simulink model "Neural_Network"  (R2013a)
settings: Solver=ode45  StartTime=0.0  StopTime=200  RelTol=1e-3
settings Model: Creator=sivom  LastModifiedBy=sivom

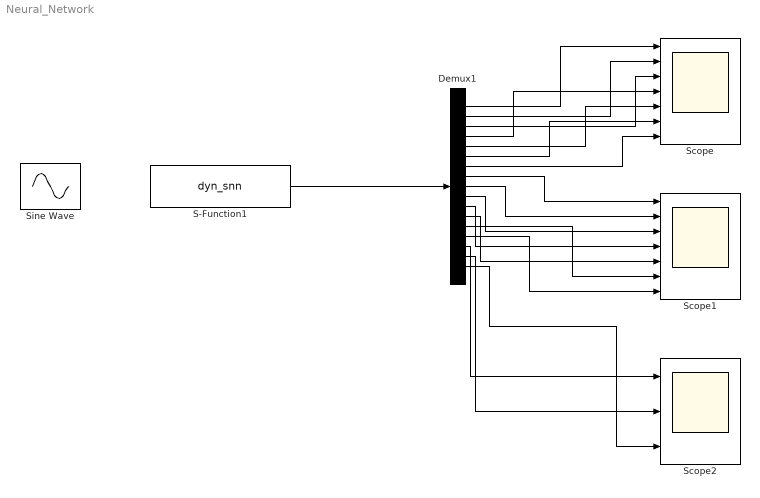
== system Neural_Network ==
  Demux1 : Demux  Outputs=17
  S-Function1 : S-Function  FunctionName=dyn_snn  EnableBusSupport=off
  Scope : Scope  NumInputPorts=7
      settings: TimeRange=50  YMin=-1.5~-1~-5~-5~-5~-5~-5  YMax=3~1~5~5~5~5~5
  Scope1 : Scope  NumInputPorts=7
      settings: TimeRange=50  YMin=-1.5~-1~-5~-5~-5~-5~-5  YMax=3~1~5~5~5~5~5
  Scope2 : Scope  NumInputPorts=3
      settings: TimeRange=50  YMin=-1.5~-1~-5  YMax=3~1~5  SaveName=ScopeData2
  Sine Wave : Sin  SampleTime=0
  wires:
  Demux1/1 -> Scope/1
  Demux1/2 -> Scope/2
  Demux1/3 -> Scope/3
  Demux1/4 -> Scope/4
  Demux1/5 -> Scope/5
  Demux1/6 -> Scope/6
  Demux1/7 -> Scope/7
  Demux1/8 -> Scope1/1
  Demux1/9 -> Scope1/2
  Demux1/10 -> Scope1/3
  Demux1/11 -> Scope1/4
  Demux1/12 -> Scope1/5
  Demux1/13 -> Scope1/6
  Demux1/14 -> Scope1/7
  Demux1/15 -> Scope2/1
  Demux1/16 -> Scope2/2
  Demux1/17 -> Scope2/3
  S-Function1/1 -> Demux1/1
